simulink model "TRS_Control_twincat_R2019a"  (R2019a)
settings: Solver=FixedStepDiscrete  StartTime=0.0  StopTime=10.0  FixedStep=0.01  RelTol=1e-3
values from neighbouring files (symbols this model uses):
  K2 = K(:,1:end-2)    [Linear_model_control.m]
  Ki = K(:,7:end)    [Linear_model_control.m]
  Ts = 10 * 10^(-3)    (= 0.01)    [Linear_model_control.m]
undefined symbols (not defined in the file or in its folder): Cd, Gamma, Ko, Phi
libraries: simulink_extras x2
settings Model: SimulationMode=external  Creator=e0371305  LastModifiedBy=jerek
settings DataIOCC: ReturnWorkspaceOutputs=off
settings OptimizationCC: LocalBlockOutputs=off
settings DebuggingCC: ArithmeticOperatorsInVariantConditions=warning
settings SFSimCC: SimUseLocalCustomCode=off
settings RTWCC: Description=TwinCAT Target  SystemTargetFile=TwinCAT.tlc  GenCodeOnly=on  MakeCommand=make_tct  TemplateMakefile=tct_msbuild.tmf  GenerateReport=on  RTWUseLocalCustomCode=off  TargetLang=C++
settings CodeAppCC: StateflowObjectComments=on
settings STFCustomTargetCC: TargetLangStandard=C++03 (ISO)  CompOptLevelCompliant=on  MATLABClassNameForMDSCustomization=Simulink.SoftwareTarget.TargetSpecificTriggerConfigurationBase  SystemTargetFile=TwinCAT.tlc

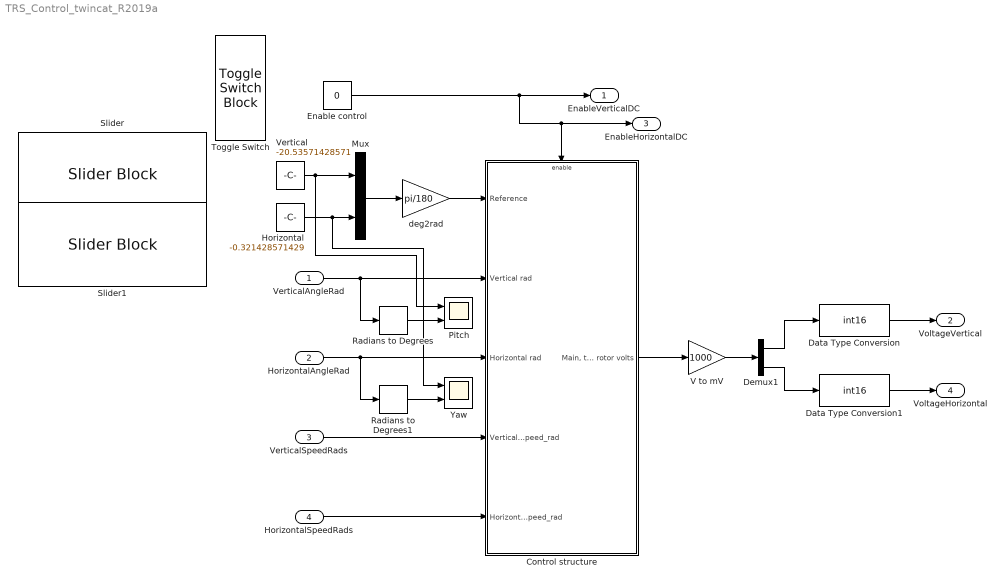
== system TRS_Control_twincat_R2019a ==
  VerticalAngleRad : Inport  OutDataTypeStr=double
  HorizontalAngleRad : Inport  Port=2  OutDataTypeStr=double
  VerticalSpeedRads : Inport  Port=3
  HorizontalSpeedRads : Inport  Port=4
  Control structure : Subsystem
  Data Type Conversion : DataTypeConversion  OutDataTypeStr=int16
  Data Type Conversion1 : DataTypeConversion  OutDataTypeStr=int16
  Demux1 : Demux  Outputs=2
  Enable control : Constant  Value=0  OutDataTypeStr=boolean
  Horizontal : Constant  Value=-0.321428571429
  Mux : Mux  Inputs=2
  Pitch : Scope  NumInputPorts=2
  Radians to Degrees : simulink_extras/Transformations/Radians to Degrees
  Radians to Degrees1 : simulink_extras/Transformations/Radians to Degrees
  Slider : SliderBlock  ScaleMin=-50  ScaleMax=0  WebBlockId=284
  Slider1 : SliderBlock  ScaleMin=-90  ScaleMax=90  WebBlockId=286
  Toggle Switch : ToggleSwitchBlock  WebBlockId=285
      settings: Values={{'Off', 'On'}, [0 1]}
  V to mV : Gain  Gain=1000
  Vertical : Constant  Value=-20.53571428571
  Yaw : Scope  NumInputPorts=2
  deg2rad : Gain  Gain=pi/180
  EnableVerticalDC : Outport  OutDataTypeStr=boolean
  VoltageVertical : Outport  Port=2
  EnableHorizontalDC : Outport  Port=3  OutDataTypeStr=boolean
  VoltageHorizontal : Outport  Port=4
  wires:
  Enable control/1 -> Control structure/Enable, EnableHorizontalDC/1, EnableVerticalDC/1
  Data Type Conversion/1 -> VoltageVertical/1
  Demux1/1 -> Data Type Conversion/1
  Data Type Conversion1/1 -> VoltageHorizontal/1
  Demux1/2 -> Data Type Conversion1/1
  Control structure/1("Main, tail rotor volts") -> V to mV/1
  Mux/1 -> deg2rad/1
  Vertical/1 -> Pitch/1, Mux/1
  Horizontal/1 -> Yaw/1, Mux/2
  deg2rad/1 -> Control structure/1(Reference)
  VerticalAngleRad/1 -> Control structure/2(Vertical rad), Radians to Degrees/1
  HorizontalAngleRad/1 -> Radians to Degrees1/1, Control structure/3(Horizontal rad)
  VerticalSpeedRads/1 -> Control structure/4(VerticalSpeed_rad)
  HorizontalSpeedRads/1 -> Control structure/5(HorizontalSpeed_rad)
  V to mV/1 -> Demux1/1
  Radians to Degrees/1 -> Pitch/2
  Radians to Degrees1/1 -> Yaw/2

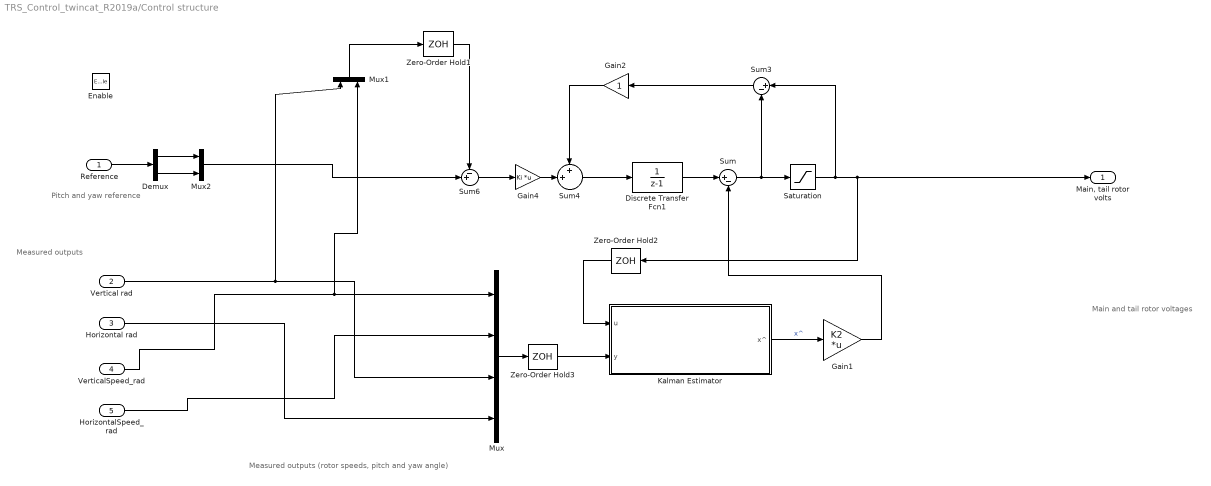
== system TRS_Control_twincat_R2019a/Control structure ==
  note: Main and tail rotor voltages
  note: Pitch and yaw reference
  note: Measured outputs (rotor speeds, pitch and yaw angle)
  note: Measured outputs
  Reference : Inport
  Vertical rad : Inport  Port=2
  Horizontal rad : Inport  Port=3
  VerticalSpeed_rad : Inport  Port=4
  HorizontalSpeed_rad : Inport  Port=5
  Enable : EnablePort  StatesWhenEnabling=reset
  Demux : Demux  Outputs=2
  Discrete Transfer Fcn1 : DiscreteTransferFcn  Denominator=[1 -1]  SampleTime=Ts
  Gain1 : Gain  Gain=K2  Multiplication=Matrix(K*u) (u vector)
  Gain2 : Gain
  Gain4 : Gain  Gain=Ki  Multiplication=Matrix(K*u) (u vector)
  Kalman Estimator : Subsystem
  Mux : Mux
  Mux1 : Mux  Inputs=2
  Mux2 : Mux  Inputs=2
  Saturation : Saturate  UpperLimit=18  LowerLimit=-18
  Sum : Sum  Inputs=|+-
  Sum3 : Sum  Inputs=|+-
  Sum4 : Sum  Inputs=++|
  Sum6 : Sum  Inputs=-+|
  Zero-Order Hold1 : ZeroOrderHold  SampleTime=Ts
  Zero-Order Hold2 : ZeroOrderHold  SampleTime=Ts
  Zero-Order Hold3 : ZeroOrderHold  SampleTime=Ts
  "Main, tail rotor volts" : Outport
  wires:
  Reference/1 -> Demux/1
  Demux/1 -> Mux2/1
  Demux/2 -> Mux2/2
  Vertical rad/1 -> Mux/3, Mux1/1
  Horizontal rad/1 -> Mux/4
  VerticalSpeed_rad/1 -> Mux1/2, Mux/1
  HorizontalSpeed_rad/1 -> Mux/2
  Kalman Estimator/1(x^) -> Gain1/1  "x^"
  Gain4/1 -> Sum4/2
  Mux2/1 -> Sum6/2
  Sum6/1 -> Gain4/1
  Sum4/1 -> Discrete Transfer Fcn1/1
  Saturation/1 -> Zero-Order Hold2/1, "Main, tail rotor volts"/1, Sum3/1
  Sum3/1 -> Gain2/1
  Gain2/1 -> Sum4/1
  Sum/1 -> Sum3/2, Saturation/1
  Discrete Transfer Fcn1/1 -> Sum/1
  Gain1/1 -> Sum/2
  Mux1/1 -> Zero-Order Hold1/1
  Zero-Order Hold1/1 -> Sum6/1
  Zero-Order Hold2/1 -> Kalman Estimator/1(u)
  Mux/1 -> Zero-Order Hold3/1
  Zero-Order Hold3/1 -> Kalman Estimator/2(y)

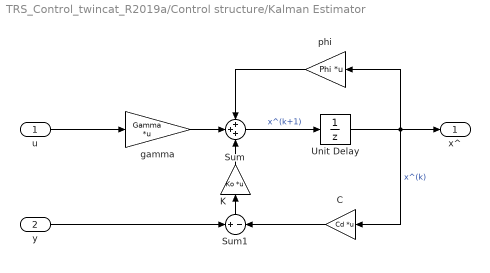
== system TRS_Control_twincat_R2019a/Control structure/Kalman Estimator ==
  u : Inport
  y : Inport  Port=2
  C : Gain  Gain=Cd  Multiplication=Matrix(K*u)  SaturateOnIntegerOverflow=on  OutDataTypeStr=Inherit: Same as input  ParamDataTypeStr=Inherit: Same as input
  K : Gain  Gain=Ko  Multiplication=Matrix(K*u)  SaturateOnIntegerOverflow=on  OutDataTypeStr=Inherit: Same as input  ParamDataTypeStr=Inherit: Same as input
  Sum : Sum  Inputs=+++  SaturateOnIntegerOverflow=on
  Sum1 : Sum  Inputs=+-  SaturateOnIntegerOverflow=on
  Unit Delay : UnitDelay  SampleTime=Ts
  gamma : Gain  Gain=Gamma  Multiplication=Matrix(K*u)  SaturateOnIntegerOverflow=on  OutDataTypeStr=Inherit: Same as input  ParamDataTypeStr=Inherit: Same as input
  phi : Gain  Gain=Phi  Multiplication=Matrix(K*u)  SaturateOnIntegerOverflow=on  OutDataTypeStr=Inherit: Same as input  ParamDataTypeStr=Inherit: Same as input
  x^ : Outport
  wires:
  K/1 -> Sum/3
  C/1 -> Sum1/2
  y/1 -> Sum1/1
  Sum1/1 -> K/1
  gamma/1 -> Sum/2
  phi/1 -> Sum/1
  Unit Delay/1 -> C/1, x^/1, phi/1  "x^(k)"
  Sum/1 -> Unit Delay/1  "x^(k+1)"
  u/1 -> gamma/1
